simulink model "marypsk_ADM"  (Simulink 8.1)
settings: Solver=ode45  StartTime=0.0  StopTime=5000  RelTol=1e-3
undefined symbols (not defined in the file): i
libraries: commsink2 x3, commdigbbndam3 x2, commchan3 x1, commrandsrc2 x1
settings Model: Creator=mrinal  LastModifiedBy=Karan
settings OptimizationCC: InitFltsAndDblsToZero=on
settings DebuggingCC: SaveWithParameterizedLinksMsg=none  SignalResolutionControl=TryResolveAllWithWarning  MultiTaskDSMMsg=warning  MultiTaskCondExecSysMsg=none  FcnCallInpInsideContextMsg=EnableAllAsWarning  StrictBusMsg=None
settings RTWCC: IncludeERTFirstTime=on
settings GRTTargetCC: TargetFcnLib=ansi_tfl_tmw.mat

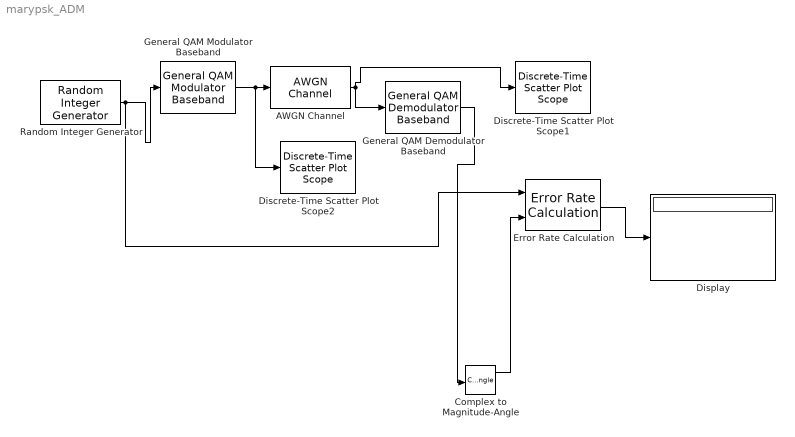
== system marypsk_ADM ==
  AWGN Channel : commchan3/AWGN Channel  InputProcessing=Inherited (this choice will be removed - see release notes)  seed=67  noiseMode="Signal to noise ratio  (SNR)"  EbNodB=4  EsNodB=10  SNRdB=20  bitsPerSym=1  Ps=1  Tsym=1  variance=1
  Complex to Magnitude-Angle : ComplexToMagnitudeAngle
  Discrete-Time Scatter Plot Scope1 : commsink2/Discrete-Time Scatter Plot Scope  Tag=ScatterPlot  sampPerSymb=1  offsetEye=0  numTraces=40  numNewFrames=10  LineMarkers=.  LineColors=[0 0 0]  fading=on  render=on  AxisGrid=off  xMin=-1.5  xMax=1.5  yMin=-1.5  yMax=1.5  inphaseLabel=In-phase Amplitude  quadratureLabel=Quadrature Amplitude  openScopeAtSimStart=on  FrameNumber=off  FigPos=[360 140 560 560]  figTitle=Scatter Plot  numLinesMax=8  block_type_=scatter
  Discrete-Time Scatter Plot Scope2 : commsink2/Discrete-Time Scatter Plot Scope  Tag=ScatterPlot  sampPerSymb=1  offsetEye=0  numTraces=40  numNewFrames=10  LineMarkers=.  LineColors=b  fading=on  render=on  AxisGrid=off  xMin=-1.5  xMax=1.5  yMin=-1.5  yMax=1.5  inphaseLabel=In-phase Amplitude  quadratureLabel=Quadrature Amplitude  openScopeAtSimStart=on  FrameNumber=off  FigPos=[360 140 560 560]  figTitle=Scatter Plot  numLinesMax=8  block_type_=scatter
  Display : Display
  Error Rate Calculation : commsink2/Error Rate Calculation  N=0  st_delay=0  cp_mode=Entire frame  subframe=[]  PMode=Port  WsName=ErrorVec  RsMode2=off  stop=off  numErr=100  maxBits=1e6
  General QAM Demodulator Baseband : commdigbbndam3/General QAM Demodulator Baseband  SigCon=[exp(2*pi*i*[0:63]/64)]  OutType=Integer  DecType=Hard decision  VarSource=Dialog  Variance=1  outDtypeBit=Inherit via internal rule  outDtype=Inherit via internal rule  roundingMode=Floor  overflowMode=Wrap  sigConstWordLen=16  accum1WordLen=32  accum1FracLen=30  prodInWordLen=32  prodInFracLen=30  prodOutWordLen=32  prodOutFracLen=30  accum2WordLen=32  accum2FracLen=30  accum3WordLen=32  accum3FracLen=30  nsiWordLen=32  nsiFracLen=30  invn0WordLen=16  invn0FracLen=8  outputWordLen=32  outputFracLen=30
  General QAM Modulator Baseband : commdigbbndam3/General QAM Modulator Baseband  SigCon=[exp(2*pi*i*[0:63]/64)]  outDtype=double  outWordLen=16  outUDDataType=sfix(16)  outFracLenMode=Best precision  outFracLen=15
  Random Integer Generator : commrandsrc2/Random Integer Generator  mul=64  seed=37  Ts=1  frameBased=on  sampPerFrame=8  orient=off  outDataType=double
  wires:
  Random Integer Generator/1 -> Error Rate Calculation/1, General QAM Modulator Baseband/1
  General QAM Demodulator Baseband/1 -> Complex to Magnitude-Angle/1
  AWGN Channel/1 -> Discrete-Time Scatter Plot Scope1/1, General QAM Demodulator Baseband/1
  Complex to Magnitude-Angle/1 -> Error Rate Calculation/2
  General QAM Modulator Baseband/1 -> Discrete-Time Scatter Plot Scope2/1, AWGN Channel/1
  Error Rate Calculation/1 -> Display/1
